simulink model "HSV_WithoutBackgroundRemove_Threshoding"  (R2016a)
settings: Solver=VariableStepAuto  StartTime=0.0  StopTime=10.0  RelTol=1e-3
undefined symbols (not defined in the file): Rec, SDTV
libraries: visionsinks x3, visionconversions x1, visionsources x1
settings Model: Creator=YASARA  LastModifiedBy=YASARA

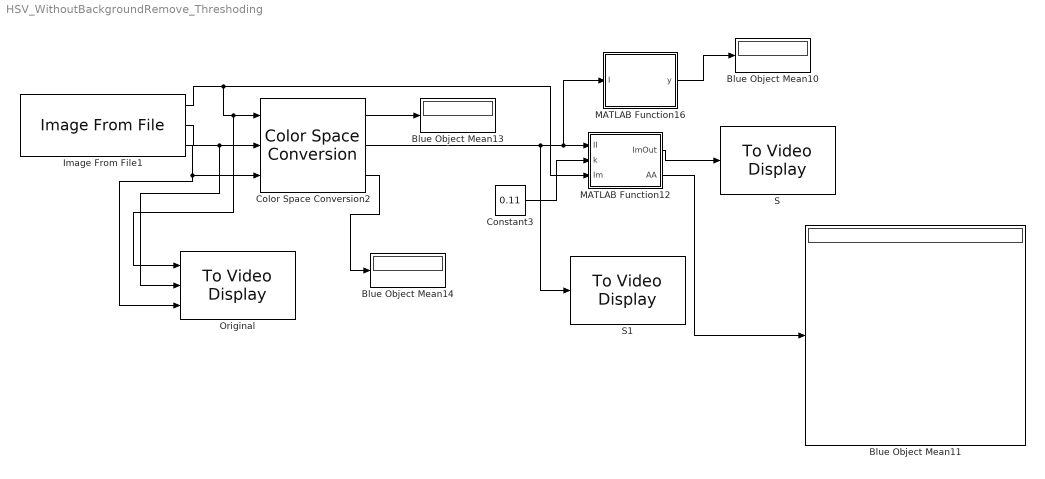
== system HSV_WithoutBackgroundRemove_Threshoding ==
  Blue Object Mean{10..11,13..14} (4 alike) : Display
  Color Space Conversion2 : visionconversions/Color Space  Conversion  conversion=Obsolete  conversionActive=R'G'B' to HSV  wp_str=D65  rec=Rec. 601 (SDTV)  sys=1125/60/2:1  imagePorts=Separate color signals
  Constant3 : Constant  Value=0.11  OutDataTypeStr=double
  Image From File1 : visionsources/Image From File  Tag=vipblks_nd  FileName=C:\Users\YASARA\Desktop\New folder (3)\Testing\Stem_Leaf\Resolution1\DSC_1324.JPG  imagePorts=Separate color signals  Ts=1  ImageDataType=double  Signed=on  WordLength=16  sdImageDataType=uint(8)  FractionLengthMode=User-defined  FractionLength=15  OutPortLabels=R|G|B
  MATLAB Function12 : MATLAB Function  TreatAsAtomicUnit=on
  MATLAB Function16 : MATLAB Function  TreatAsAtomicUnit=on
  Original : visionsinks/To Video Display  windowSizeMode=Normal  openAtMdlStart=on  fullScreen=off  videoWindowX=252  videoWindowY=213  saveWindowSize=off  videoWindowWidth=512  videoWindowHeight=384  inputColorFormat=RGB  inputType=Obsolete  imagePorts=Separate color signals  OutputDevice=On-screen video monitor  dataOrg=Column-major  isWindowOpen=off
  S : visionsinks/To Video Display  windowSizeMode=Normal  openAtMdlStart=on  fullScreen=off  videoWindowX=252  videoWindowY=213  saveWindowSize=off  videoWindowWidth=512  videoWindowHeight=384  inputColorFormat=RGB  inputType=Obsolete  imagePorts=One multidimensional signal  OutputDevice=On-screen video monitor  dataOrg=Column-major  isWindowOpen=off
  S1 : visionsinks/To Video Display  windowSizeMode=Normal  openAtMdlStart=on  fullScreen=off  videoWindowX=252  videoWindowY=213  saveWindowSize=off  videoWindowWidth=512  videoWindowHeight=384  inputColorFormat=RGB  inputType=Obsolete  imagePorts=One multidimensional signal  OutputDevice=On-screen video monitor  dataOrg=Column-major  isWindowOpen=off
  wires:
  Image From File1/2 -> Original/2, Color Space Conversion2/2
  Color Space Conversion2/1 -> Blue Object Mean13/1
  Color Space Conversion2/2 -> S1/1, MATLAB Function16/1(I), MATLAB Function12/1(II)
  Constant3/1 -> MATLAB Function12/2(k)
  MATLAB Function12/1(ImOut) -> S/1
  Color Space Conversion2/3 -> Blue Object Mean14/1
  MATLAB Function16/1(y) -> Blue Object Mean10/1
  MATLAB Function12/2(AA) -> Blue Object Mean11/1
  Image From File1/3 -> Original/3, Color Space Conversion2/3
  Image From File1/1 -> Original/1, Color Space Conversion2/1, MATLAB Function12/3(Im)

== matlab function HSV_WithoutBackgroundRemove_Threshoding/MATLAB Function12 ==
  data: II input; ImOut output; k input; Im input; AA output
function [ImOut,AA] = fcn(II,k,Im)
I=Im;
coder.extrinsic('graythresh');
coder.extrinsic('im2bw');
level = graythresh(I);
BW = im2bw(I,level);
L=double(I);
coder.extrinsic('bwlabeln');
NUM=1;
BW2=imcomplement(BW);
[L, NUM] = bwlabeln(BW2);
area=1;
n=1;
R1=double(II);
AA=double(zeros(100,1));
i=1;
for n=1:NUM
    [r, c] = find(L==n);
    %if (max(c)~= min(c))&&(max(r)~= min(r))
    if ((max(c)-min(c))>50)&&((max(r)-min(r))>50)
        t=R1(L==n);
        AA(i)=mean(t(:));         
        if (AA(i)>k)
           R1(L==n)=0; 
           
        end
        i=i+1;
    end
end;
ImOut=R1;

== matlab function HSV_WithoutBackgroundRemove_Threshoding/MATLAB Function16 ==
  data: I input; y output
function y = fcn(I)
y=mean(I(:));
